simulink model "ThdRwRtStCshnFldTrgtPosSelc"  (R2018b)
settings: Solver=FixedStepDiscrete  StartTime=0.0  StopTime=10.0  RelTol=1e-3
undefined symbols (not defined in the file or in its folder): KeSMSw6sAcsEntryThdRwRtStCshnFldUpwdDnwdPos_Val, KeSMSw6sAcsEntryThdRwRtStCshnFldUpwdDnwdPosMax_Val, KeSMSw6sAcsEntryThdRwRtStCshnFldUpwdDnwdPosMin_Val, KeSMSw6sLugThdRwRtStCshnFldUpwdDnwdPos_Val, KeSMSw6sLugThdRwRtStCshnFldUpwdDnwdPosMax_Val, KeSMSw6sLugThdRwRtStCshnFldUpwdDnwdPosMin_Val, KeSMSwAcsEntryThdRwRtStCshnFldUpwdDnwdPos_Val, KeSMSwAcsEntryThdRwRtStCshnFldUpwdDnwdPosMax_Val, KeSMSwAcsEntryThdRwRtStCshnFldUpwdDnwdPosMin_Val, KeSMSwAcsMd53ThdRwRtFldUpwdDnwdPos_Val, KeSMSwAcsMd53ThdRwRtFldUpwdDnwdPosMax_Val, KeSMSwAcsMd53ThdRwRtFldUpwdDnwdPosMin_Val, KeSMSwLugThdRwRtStCshnFldUpwdDnwdPos_Val, KeSMSwLugThdRwRtStCshnFldUpwdDnwdPosMax_Val, KeSMSwLugThdRwRtStCshnFldUpwdDnwdPosMin_Val
libraries: TrgtPosSelcLib x4
settings Model: ModifiedHistory=2024.6.25 V2.1.0 557模式流程V1.6  Creator=sn2xws  LastModifiedBy=sn2xws
settings DataIOCC: SaveFormat=StructureWithTime
settings OptimizationCC: DefaultParameterBehavior=Inlined  EnhancedBackFolding=on  PassReuseOutputArgsAs=Individual arguments  ZeroExternalMemoryAtStartup=off  ZeroInternalMemoryAtStartup=off  OptimizeBlockOrder=speed  DifferentSizesBufferReuse=on  OptimizationCustomize=off
settings DebuggingCC: ParameterTunabilityLossMsg=error
settings SFSimCC: MATLABDynamicMemAlloc=off
settings RTWCC: SystemTargetFile=autosar.tlc  GenCodeOnly=on  TemplateMakefile=ert_default_tmf  Description=AUTOSAR  GenerateReport=on  IncludeHyperlinkInReport=on  LaunchReport=on  GenerateTraceInfo=on  GenerateTraceReport=on  GenerateTraceReportSl=on  GenerateTraceReportSf=on  GenerateTraceReportEml=on
settings CodeAppCC: ForceParamTrailComments=on  IgnoreCustomStorageClasses=off  OperatorAnnotations=on  SimulinkDataObjDesc=on  SFDataObjDesc=on  InsertBlockDesc=on
settings STFCustomTargetCC: TargetLangStandard=C99 (ISO)  MultiwordLength=256  ParMdlRefBuildCompliant=on  CompOptLevelCompliant=on  IncludeMdlTerminateFcn=off  CombineOutputUpdateFcns=on  SuppressErrorStatus=on  ERTCustomFileBanners=on  SupportNonFinite=off  SupportComplex=off  SupportContinuousTime=off  SupportNonInlinedSFcns=off  RemoveResetFunc=on  MATLABClassNameForMDSCustomization=Simulink.SoftwareTarget.ERTCustomization  AutosarCompliant=on  UseToolchainInfoCompliant=on  LookupTableObjectStructAxisOrder=2,1,3,4,...  LUTObjectStructOrderEvenSpacing=Size,Table,Breakpoints  SystemTargetFile=autosar.tlc
settings ERTTargetCC: TargetLangStandard=C99 (ISO)  ConcurrentExecutionCompliant=off  IncludeMdlTerminateFcn=off  SuppressErrorStatus=on  SupportNonFinite=off  SupportComplex=off  ModelStepFunctionPrototypeControlCompliant=off  CPPClassGenCompliant=off  AutosarCompliant=on  LookupTableObjectStructAxisOrder=2,1,3,4,...  LUTObjectStructOrderEvenSpacing=Size,Table,Breakpoints  InlinedParameterPlacement=NonHierarchical  ERTCustomFileTemplate=example_file_process.tlc  ERTFilePackagingFormat=Compact

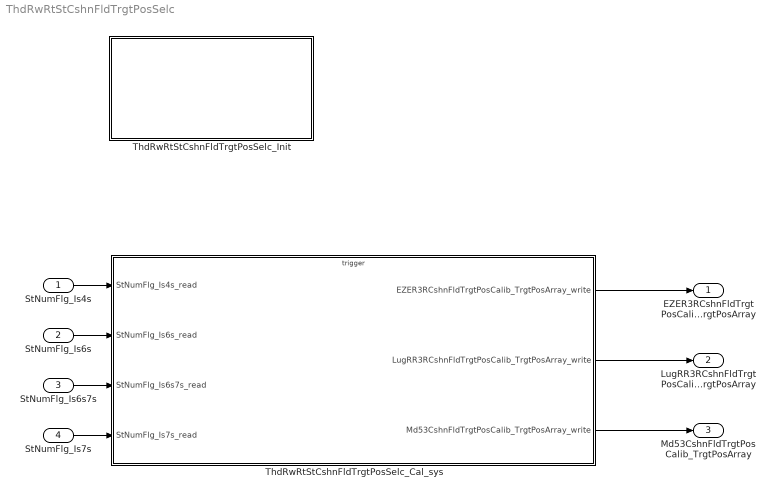
== system ThdRwRtStCshnFldTrgtPosSelc ==
  StNumFlg_Is4s : Inport  OutDataTypeStr=boolean  PortDimensions=1
  StNumFlg_Is6s : Inport  Port=2  OutDataTypeStr=boolean  PortDimensions=1
  StNumFlg_Is6s7s : Inport  Port=3  OutDataTypeStr=boolean  PortDimensions=1
  StNumFlg_Is7s : Inport  Port=4  OutDataTypeStr=boolean  PortDimensions=1
  ThdRwRtStCshnFldTrgtPosSelc_Cal_sys : Subsystem
  ThdRwRtStCshnFldTrgtPosSelc_Init : Subsystem
  EZER3RCshnFldTrgtPosCalib_TrgtPosArray : Outport  Description=|  OutDataTypeStr=uint16  PortDimensions=3
      | 0:Pos
      | 1:Max
      | 2:Min
  LugRR3RCshnFldTrgtPosCalib_TrgtPosArray : Outport  Description=|  Port=2  OutDataTypeStr=uint16  PortDimensions=3
      | 0:Pos
      | 1:Max
      | 2:Min
  Md53CshnFldTrgtPosCalib_TrgtPosArray : Outport  Description=|  Port=3  OutDataTypeStr=uint16  PortDimensions=3
      | 0:Pos
      | 1:Max
      | 2:Min
  wires:
  StNumFlg_Is4s/1 -> ThdRwRtStCshnFldTrgtPosSelc_Cal_sys/1(StNumFlg_Is4s_read)
  StNumFlg_Is6s/1 -> ThdRwRtStCshnFldTrgtPosSelc_Cal_sys/2(StNumFlg_Is6s_read)
  StNumFlg_Is6s7s/1 -> ThdRwRtStCshnFldTrgtPosSelc_Cal_sys/3(StNumFlg_Is6s7s_read)
  StNumFlg_Is7s/1 -> ThdRwRtStCshnFldTrgtPosSelc_Cal_sys/4(StNumFlg_Is7s_read)
  ThdRwRtStCshnFldTrgtPosSelc_Cal_sys/1(EZER3RCshnFldTrgtPosCalib_TrgtPosArray_write) -> EZER3RCshnFldTrgtPosCalib_TrgtPosArray/1
  ThdRwRtStCshnFldTrgtPosSelc_Cal_sys/2(LugRR3RCshnFldTrgtPosCalib_TrgtPosArray_write) -> LugRR3RCshnFldTrgtPosCalib_TrgtPosArray/1
  ThdRwRtStCshnFldTrgtPosSelc_Cal_sys/3(Md53CshnFldTrgtPosCalib_TrgtPosArray_write) -> Md53CshnFldTrgtPosCalib_TrgtPosArray/1

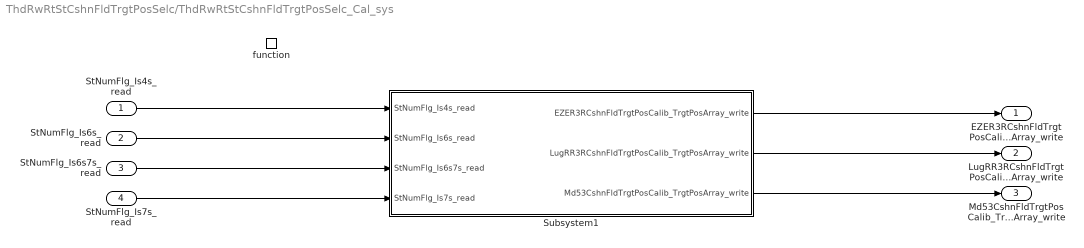
== system ThdRwRtStCshnFldTrgtPosSelc/ThdRwRtStCshnFldTrgtPosSelc_Cal_sys ==
  StNumFlg_Is4s_read : Inport
  StNumFlg_Is6s_read : Inport  Port=2
  StNumFlg_Is6s7s_read : Inport  Port=3
  StNumFlg_Is7s_read : Inport  Port=4
  function : TriggerPort  TriggerType=function-call  IsSimulinkFunction=on  FunctionName=ThdRwRtStCshnFldTrgtPosSelc_Cal  VariantControl=(inherit)
  Subsystem1 : Subsystem
  EZER3RCshnFldTrgtPosCalib_TrgtPosArray_write : Outport
      settings: EnsureOutportIsVirtual=on
  LugRR3RCshnFldTrgtPosCalib_TrgtPosArray_write : Outport  Port=2
      settings: EnsureOutportIsVirtual=on
  Md53CshnFldTrgtPosCalib_TrgtPosArray_write : Outport  Port=3
      settings: EnsureOutportIsVirtual=on
  wires:
  Subsystem1/1(EZER3RCshnFldTrgtPosCalib_TrgtPosArray_write) -> EZER3RCshnFldTrgtPosCalib_TrgtPosArray_write/1
  Subsystem1/2(LugRR3RCshnFldTrgtPosCalib_TrgtPosArray_write) -> LugRR3RCshnFldTrgtPosCalib_TrgtPosArray_write/1
  StNumFlg_Is4s_read/1 -> Subsystem1/1(StNumFlg_Is4s_read)
  StNumFlg_Is6s_read/1 -> Subsystem1/2(StNumFlg_Is6s_read)
  StNumFlg_Is6s7s_read/1 -> Subsystem1/3(StNumFlg_Is6s7s_read)
  StNumFlg_Is7s_read/1 -> Subsystem1/4(StNumFlg_Is7s_read)
  ? -> ?
  Subsystem1/3(Md53CshnFldTrgtPosCalib_TrgtPosArray_write) -> Md53CshnFldTrgtPosCalib_TrgtPosArray_write/1

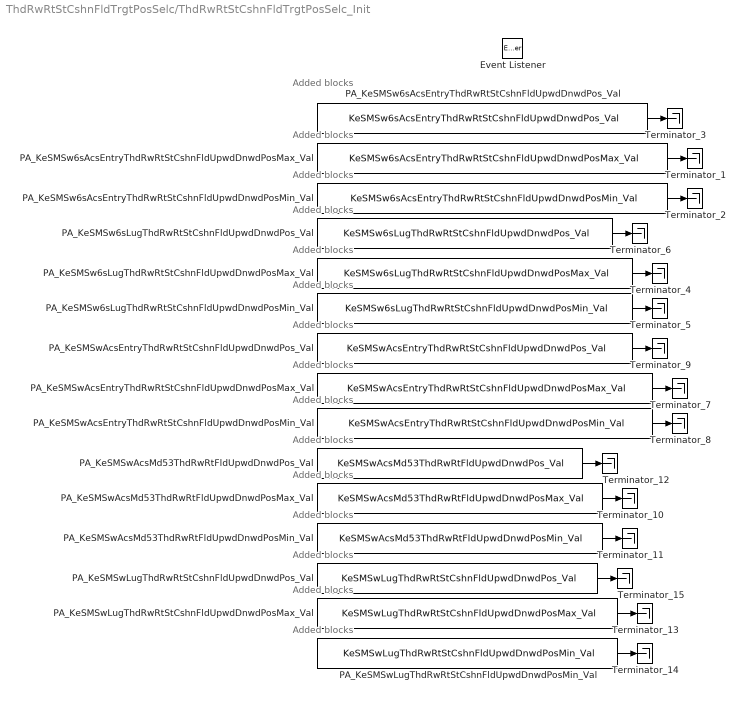
== system ThdRwRtStCshnFldTrgtPosSelc/ThdRwRtStCshnFldTrgtPosSelc_Init ==
  note: Added blocks
  note: Added blocks
  note: Added blocks
  note: Added blocks
  note: Added blocks
  note: Added blocks
  note: Added blocks
  note: Added blocks
  note: Added blocks
  note: Added blocks
  note: Added blocks
  note: Added blocks
  note: Added blocks
  note: Added blocks
  note: Added blocks
  Event Listener : EventListener  EventName=reset
  PA_KeSMSw6sAcsEntryThdRwRtStCshnFldUpwdDnwdPosMax_Val : Constant  Value=KeSMSw6sAcsEntryThdRwRtStCshnFldUpwdDnwdPosMax_Val
  PA_KeSMSw6sAcsEntryThdRwRtStCshnFldUpwdDnwdPosMin_Val : Constant  Value=KeSMSw6sAcsEntryThdRwRtStCshnFldUpwdDnwdPosMin_Val
  PA_KeSMSw6sAcsEntryThdRwRtStCshnFldUpwdDnwdPos_Val : Constant  Value=KeSMSw6sAcsEntryThdRwRtStCshnFldUpwdDnwdPos_Val
  PA_KeSMSw6sLugThdRwRtStCshnFldUpwdDnwdPosMax_Val : Constant  Value=KeSMSw6sLugThdRwRtStCshnFldUpwdDnwdPosMax_Val
  PA_KeSMSw6sLugThdRwRtStCshnFldUpwdDnwdPosMin_Val : Constant  Value=KeSMSw6sLugThdRwRtStCshnFldUpwdDnwdPosMin_Val
  PA_KeSMSw6sLugThdRwRtStCshnFldUpwdDnwdPos_Val : Constant  Value=KeSMSw6sLugThdRwRtStCshnFldUpwdDnwdPos_Val
  PA_KeSMSwAcsEntryThdRwRtStCshnFldUpwdDnwdPosMax_Val : Constant  Value=KeSMSwAcsEntryThdRwRtStCshnFldUpwdDnwdPosMax_Val
  PA_KeSMSwAcsEntryThdRwRtStCshnFldUpwdDnwdPosMin_Val : Constant  Value=KeSMSwAcsEntryThdRwRtStCshnFldUpwdDnwdPosMin_Val
  PA_KeSMSwAcsEntryThdRwRtStCshnFldUpwdDnwdPos_Val : Constant  Value=KeSMSwAcsEntryThdRwRtStCshnFldUpwdDnwdPos_Val
  PA_KeSMSwAcsMd53ThdRwRtFldUpwdDnwdPosMax_Val : Constant  Value=KeSMSwAcsMd53ThdRwRtFldUpwdDnwdPosMax_Val
  PA_KeSMSwAcsMd53ThdRwRtFldUpwdDnwdPosMin_Val : Constant  Value=KeSMSwAcsMd53ThdRwRtFldUpwdDnwdPosMin_Val
  PA_KeSMSwAcsMd53ThdRwRtFldUpwdDnwdPos_Val : Constant  Value=KeSMSwAcsMd53ThdRwRtFldUpwdDnwdPos_Val
  PA_KeSMSwLugThdRwRtStCshnFldUpwdDnwdPosMax_Val : Constant  Value=KeSMSwLugThdRwRtStCshnFldUpwdDnwdPosMax_Val
  PA_KeSMSwLugThdRwRtStCshnFldUpwdDnwdPosMin_Val : Constant  Value=KeSMSwLugThdRwRtStCshnFldUpwdDnwdPosMin_Val
  PA_KeSMSwLugThdRwRtStCshnFldUpwdDnwdPos_Val : Constant  Value=KeSMSwLugThdRwRtStCshnFldUpwdDnwdPos_Val
  Terminator_{1..15} (15 alike) : Terminator
  wires:
  PA_KeSMSw6sAcsEntryThdRwRtStCshnFldUpwdDnwdPosMax_Val/1 -> Terminator_1/1
  PA_KeSMSw6sAcsEntryThdRwRtStCshnFldUpwdDnwdPosMin_Val/1 -> Terminator_2/1
  PA_KeSMSw6sAcsEntryThdRwRtStCshnFldUpwdDnwdPos_Val/1 -> Terminator_3/1
  PA_KeSMSw6sLugThdRwRtStCshnFldUpwdDnwdPosMax_Val/1 -> Terminator_4/1
  PA_KeSMSw6sLugThdRwRtStCshnFldUpwdDnwdPosMin_Val/1 -> Terminator_5/1
  PA_KeSMSw6sLugThdRwRtStCshnFldUpwdDnwdPos_Val/1 -> Terminator_6/1
  PA_KeSMSwAcsEntryThdRwRtStCshnFldUpwdDnwdPosMax_Val/1 -> Terminator_7/1
  PA_KeSMSwAcsEntryThdRwRtStCshnFldUpwdDnwdPosMin_Val/1 -> Terminator_8/1
  PA_KeSMSwAcsEntryThdRwRtStCshnFldUpwdDnwdPos_Val/1 -> Terminator_9/1
  PA_KeSMSwAcsMd53ThdRwRtFldUpwdDnwdPosMax_Val/1 -> Terminator_10/1
  PA_KeSMSwAcsMd53ThdRwRtFldUpwdDnwdPosMin_Val/1 -> Terminator_11/1
  PA_KeSMSwAcsMd53ThdRwRtFldUpwdDnwdPos_Val/1 -> Terminator_12/1
  PA_KeSMSwLugThdRwRtStCshnFldUpwdDnwdPosMax_Val/1 -> Terminator_13/1
  PA_KeSMSwLugThdRwRtStCshnFldUpwdDnwdPosMin_Val/1 -> Terminator_14/1
  PA_KeSMSwLugThdRwRtStCshnFldUpwdDnwdPos_Val/1 -> Terminator_15/1

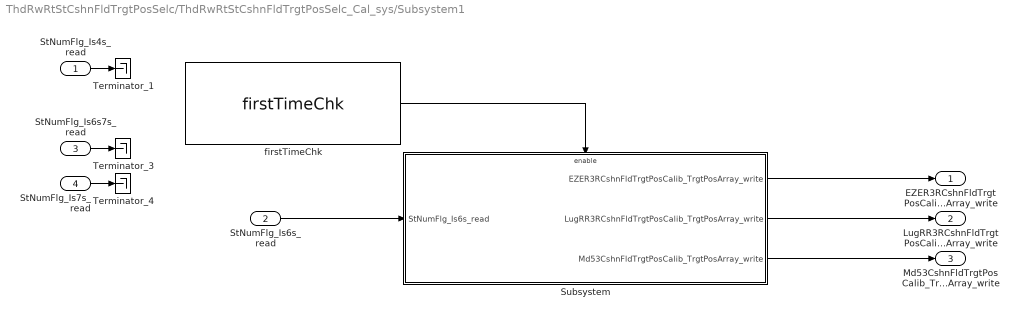
== system ThdRwRtStCshnFldTrgtPosSelc/ThdRwRtStCshnFldTrgtPosSelc_Cal_sys/Subsystem1 ==
  StNumFlg_Is4s_read : Inport
  StNumFlg_Is6s_read : Inport  Port=2
  StNumFlg_Is6s7s_read : Inport  Port=3
  StNumFlg_Is7s_read : Inport  Port=4
  Subsystem : Subsystem
  Terminator_1 : Terminator
  Terminator_3 : Terminator
  Terminator_4 : Terminator
  firstTimeChk : TrgtPosSelcLib/firstTimeChk  SystemSampleTime=-1
  EZER3RCshnFldTrgtPosCalib_TrgtPosArray_write : Outport
      settings: EnsureOutportIsVirtual=on
  LugRR3RCshnFldTrgtPosCalib_TrgtPosArray_write : Outport  Port=2
      settings: EnsureOutportIsVirtual=on
  Md53CshnFldTrgtPosCalib_TrgtPosArray_write : Outport  Port=3
      settings: EnsureOutportIsVirtual=on
  wires:
  firstTimeChk/1 -> Subsystem/Enable
  StNumFlg_Is6s7s_read/1 -> Terminator_3/1
  StNumFlg_Is4s_read/1 -> Terminator_1/1
  StNumFlg_Is7s_read/1 -> Terminator_4/1
  Subsystem/1(EZER3RCshnFldTrgtPosCalib_TrgtPosArray_write) -> EZER3RCshnFldTrgtPosCalib_TrgtPosArray_write/1
  StNumFlg_Is6s_read/1 -> Subsystem/1(StNumFlg_Is6s_read)
  Subsystem/2(LugRR3RCshnFldTrgtPosCalib_TrgtPosArray_write) -> LugRR3RCshnFldTrgtPosCalib_TrgtPosArray_write/1
  Subsystem/3(Md53CshnFldTrgtPosCalib_TrgtPosArray_write) -> Md53CshnFldTrgtPosCalib_TrgtPosArray_write/1

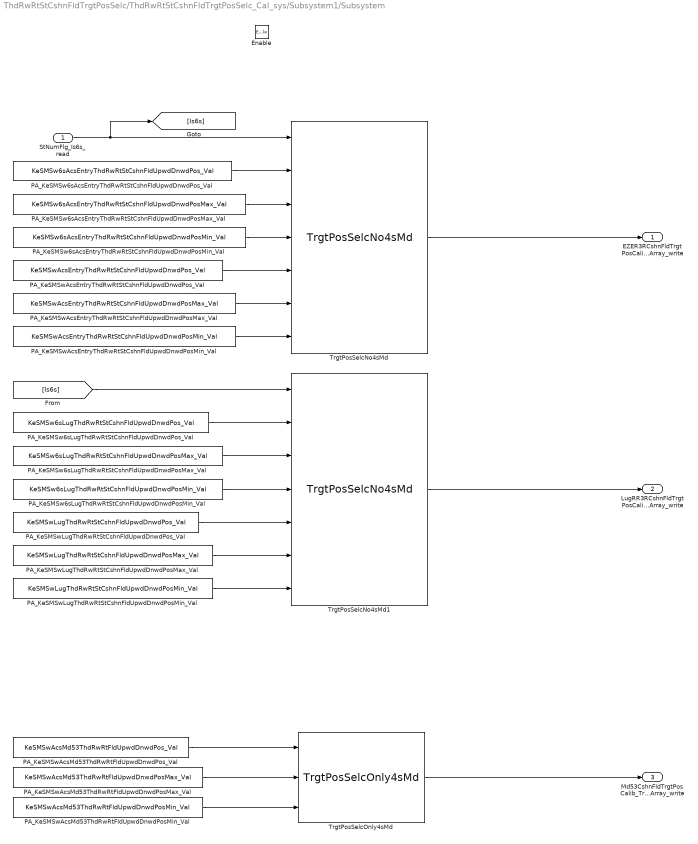
== system ThdRwRtStCshnFldTrgtPosSelc/ThdRwRtStCshnFldTrgtPosSelc_Cal_sys/Subsystem1/Subsystem ==
  StNumFlg_Is6s_read : Inport
  Enable : EnablePort
  PA_KeSMSw6sAcsEntryThdRwRtStCshnFldUpwdDnwdPosMax_Val : Constant  Value=KeSMSw6sAcsEntryThdRwRtStCshnFldUpwdDnwdPosMax_Val
  PA_KeSMSw6sAcsEntryThdRwRtStCshnFldUpwdDnwdPosMin_Val : Constant  Value=KeSMSw6sAcsEntryThdRwRtStCshnFldUpwdDnwdPosMin_Val
  PA_KeSMSw6sAcsEntryThdRwRtStCshnFldUpwdDnwdPos_Val : Constant  Value=KeSMSw6sAcsEntryThdRwRtStCshnFldUpwdDnwdPos_Val
  PA_KeSMSw6sLugThdRwRtStCshnFldUpwdDnwdPosMax_Val : Constant  Value=KeSMSw6sLugThdRwRtStCshnFldUpwdDnwdPosMax_Val
  PA_KeSMSw6sLugThdRwRtStCshnFldUpwdDnwdPosMin_Val : Constant  Value=KeSMSw6sLugThdRwRtStCshnFldUpwdDnwdPosMin_Val
  PA_KeSMSw6sLugThdRwRtStCshnFldUpwdDnwdPos_Val : Constant  Value=KeSMSw6sLugThdRwRtStCshnFldUpwdDnwdPos_Val
  PA_KeSMSwAcsEntryThdRwRtStCshnFldUpwdDnwdPosMax_Val : Constant  Value=KeSMSwAcsEntryThdRwRtStCshnFldUpwdDnwdPosMax_Val
  PA_KeSMSwAcsEntryThdRwRtStCshnFldUpwdDnwdPosMin_Val : Constant  Value=KeSMSwAcsEntryThdRwRtStCshnFldUpwdDnwdPosMin_Val
  PA_KeSMSwAcsEntryThdRwRtStCshnFldUpwdDnwdPos_Val : Constant  Value=KeSMSwAcsEntryThdRwRtStCshnFldUpwdDnwdPos_Val
  PA_KeSMSwAcsMd53ThdRwRtFldUpwdDnwdPosMax_Val : Constant  Value=KeSMSwAcsMd53ThdRwRtFldUpwdDnwdPosMax_Val
  PA_KeSMSwAcsMd53ThdRwRtFldUpwdDnwdPosMin_Val : Constant  Value=KeSMSwAcsMd53ThdRwRtFldUpwdDnwdPosMin_Val
  PA_KeSMSwAcsMd53ThdRwRtFldUpwdDnwdPos_Val : Constant  Value=KeSMSwAcsMd53ThdRwRtFldUpwdDnwdPos_Val
  PA_KeSMSwLugThdRwRtStCshnFldUpwdDnwdPosMax_Val : Constant  Value=KeSMSwLugThdRwRtStCshnFldUpwdDnwdPosMax_Val
  PA_KeSMSwLugThdRwRtStCshnFldUpwdDnwdPosMin_Val : Constant  Value=KeSMSwLugThdRwRtStCshnFldUpwdDnwdPosMin_Val
  PA_KeSMSwLugThdRwRtStCshnFldUpwdDnwdPos_Val : Constant  Value=KeSMSwLugThdRwRtStCshnFldUpwdDnwdPos_Val
  TrgtPosSelcNo4sMd : TrgtPosSelcLib/TrgtPosSelcNo4sMd  SystemSampleTime=-1
  TrgtPosSelcNo4sMd1 : TrgtPosSelcLib/TrgtPosSelcNo4sMd  SystemSampleTime=-1
  TrgtPosSelcOnly4sMd : TrgtPosSelcLib/TrgtPosSelcOnly4sMd  SystemSampleTime=-1
  EZER3RCshnFldTrgtPosCalib_TrgtPosArray_write : Outport
      settings: EnsureOutportIsVirtual=on
  LugRR3RCshnFldTrgtPosCalib_TrgtPosArray_write : Outport  Port=2
      settings: EnsureOutportIsVirtual=on
  Md53CshnFldTrgtPosCalib_TrgtPosArray_write : Outport  Port=3
      settings: EnsureOutportIsVirtual=on
  wires:
  StNumFlg_Is6s_read/1 -> [Is6s], TrgtPosSelcNo4sMd/1
  TrgtPosSelcNo4sMd/1 -> EZER3RCshnFldTrgtPosCalib_TrgtPosArray_write/1
  TrgtPosSelcNo4sMd1/1 -> LugRR3RCshnFldTrgtPosCalib_TrgtPosArray_write/1
  PA_KeSMSw6sAcsEntryThdRwRtStCshnFldUpwdDnwdPosMax_Val/1 -> TrgtPosSelcNo4sMd/3
  PA_KeSMSw6sAcsEntryThdRwRtStCshnFldUpwdDnwdPos_Val/1 -> TrgtPosSelcNo4sMd/2
  PA_KeSMSw6sAcsEntryThdRwRtStCshnFldUpwdDnwdPosMin_Val/1 -> TrgtPosSelcNo4sMd/4
  PA_KeSMSwAcsEntryThdRwRtStCshnFldUpwdDnwdPosMax_Val/1 -> TrgtPosSelcNo4sMd/6
  PA_KeSMSwAcsEntryThdRwRtStCshnFldUpwdDnwdPosMin_Val/1 -> TrgtPosSelcNo4sMd/7
  PA_KeSMSwAcsEntryThdRwRtStCshnFldUpwdDnwdPos_Val/1 -> TrgtPosSelcNo4sMd/5
  [Is6s] -> TrgtPosSelcNo4sMd1/1
  PA_KeSMSw6sLugThdRwRtStCshnFldUpwdDnwdPosMax_Val/1 -> TrgtPosSelcNo4sMd1/3
  PA_KeSMSw6sLugThdRwRtStCshnFldUpwdDnwdPos_Val/1 -> TrgtPosSelcNo4sMd1/2
  PA_KeSMSw6sLugThdRwRtStCshnFldUpwdDnwdPosMin_Val/1 -> TrgtPosSelcNo4sMd1/4
  PA_KeSMSwLugThdRwRtStCshnFldUpwdDnwdPosMin_Val/1 -> TrgtPosSelcNo4sMd1/7
  PA_KeSMSwLugThdRwRtStCshnFldUpwdDnwdPosMax_Val/1 -> TrgtPosSelcNo4sMd1/6
  PA_KeSMSwLugThdRwRtStCshnFldUpwdDnwdPos_Val/1 -> TrgtPosSelcNo4sMd1/5
  PA_KeSMSwAcsMd53ThdRwRtFldUpwdDnwdPos_Val/1 -> TrgtPosSelcOnly4sMd/1
  PA_KeSMSwAcsMd53ThdRwRtFldUpwdDnwdPosMax_Val/1 -> TrgtPosSelcOnly4sMd/2
  PA_KeSMSwAcsMd53ThdRwRtFldUpwdDnwdPosMin_Val/1 -> TrgtPosSelcOnly4sMd/3
  TrgtPosSelcOnly4sMd/1 -> Md53CshnFldTrgtPosCalib_TrgtPosArray_write/1
